simulink subsystem "VehicleElectroThermal"  (R2023a)
settings: Solver=VariableStepAuto  StartTime=0.0  StopTime=10.0  RelTol=1e-3
undefined symbols (not defined in the file): battery, cabin_T_init, coolant_pipe_D, coolant_valve_D_ratio_max, coolant_valve_D_ratio_min, coolant_valve_displacement, vehicleThermal
libraries: fl_lib x199, nesl_utility x54, SimscapeFluids_lib x15, ee_lib x9, sdl_lib x8, slpidlib x3, simulink x2, EmotorLib x2, BatteryCurrentManagement x1
(part 4 of 6)

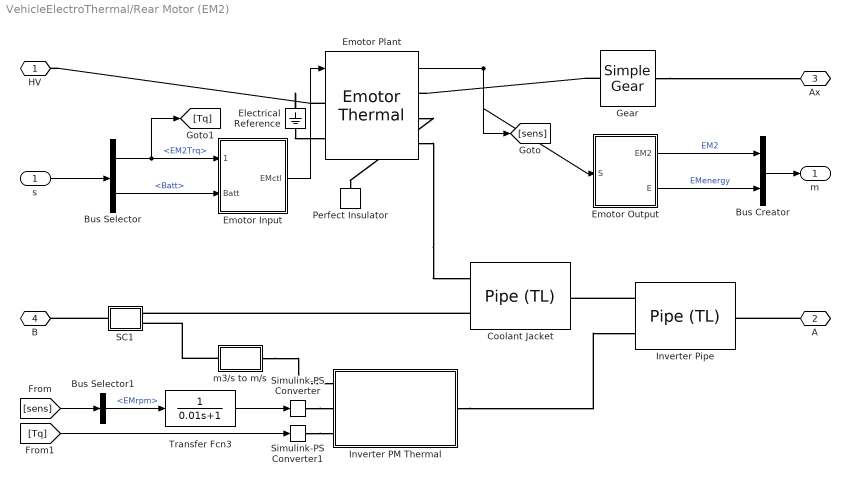
== system VehicleElectroThermal/Rear Motor (EM2) ==
  s : Inport
  Bus Creator : BusCreator  Inputs=2
  Bus Selector : BusSelector  OutputSignals=EM2Trq,Batt
  Bus Selector1 : BusSelector  OutputSignals=EMrpm
  Coolant Jacket : SimscapeFluids_lib/Thermal Liquid/Pipes & Fittings/Pipe (TL)  dynamic_compressibility=1  inertia=0  num_segments=1  pipe_length=0.4 m  cross_section_geometry=fluids.thermal_liquid.pipes_fittings.enum.CrossSectionGeometry.Custom  pipe_diameter=0.1 m  pipe_inner_diameter=0.05 m  pipe_outer_diameter=0.1 m  pipe_width=0.1 m  pipe_height=0.1 m  pipe_major_axis=0.1 m  pipe_minor_axis=0.05 m  pipe_side=0.1 m  pipe_angle=30 deg  area=4 * pi * vehicleThermal.coolant_channel_D^2 / 4 m^2  Dh=vehicleThermal.coolant_channel_D m  wall_spec=1  wall_compliance=1.2e-6 m/MPa  wall_time_constant=0.01 s  elevation_spec=foundation.enum.constant_variable.constant  elevation_gain=0 m  g=9.81 m/s^2  pressure_loss_spec=1  local_pressure_loss_spec=fluids.thermal_liquid.pipes_fittings.enum.LocalLossSpec.AggregateLength  length_add=20 * vehicleThermal.coolant_channel_D * 4 m  loss_coefficient=0.1  roughness_spec=fluids.thermal_liquid.pipes_fittings.enum.RoughnessSpec.Custom  roughness=1.5e-5 m  Re_friction_TLU=[ 400 1000 1.5e+3 3e+3 4e+3 6e+3 1e+4 2e+4 4e+4 6e+4 1e+5 1e+8 ]  friction_factor_TLU=[ 0.264 0.112 0.07099999999999999 0.0417 0.0387 0.0268 0.025 0.0232 0.0226 0.022 0.0214 0.0214 ]  shape_factor=64  Re_lam=100  Re_tur=500  mdot_nominal=[ 0.1 1 ] kg/s  p_diff_nominal=[ 0.001 0.01 ] MPa  mdot_threshold=1e-6 kg/s  heat_transfer_spec=4  mdot_nominal_heat=[ 0.1 1 ] kg/s  T_in_nominal=[ 293.15 293.15 ] K  T_out_nominal=[ 300 300 ] K  p_in_nominal_heat=[ 0.101325 0.101325 ] MPa  T_wall_nominal=[ 303.15 303.15 ] K  a_coeff=0.3  b_Re_power=0.8  c_Pr_power=0.33  Nu_lam=3.66  Re_Colburn_TLU=[ 100 150 1000 ]  Colburn_factor_TLU=[ 0.019 0.013 0.002 ]  Re_Nu_TLU=[ 100 150 1000 ]  Pr_Nu_TLU=[ 1 10 ]  Nu_TLU=[ 3.72 4.21; 3.75 4.44; 4.21 7.15 ]  p0_vec=vehicleThermal.coolant_p_init MPa  T0_vec=vehicleThermal.coolant_T_init K  mdot0=0.1 kg/s
  Electrical Reference : fl_lib/Electrical/Electrical Elements/Electrical Reference
  Emotor Input : Subsystem
  Emotor Output : Subsystem
  Emotor Plant : EmotorLib/Emotor Thermal  InitTemp=vehicleThermal.coolant_T_init  IronSpHeat=electricDrive.IronSpHeat  CopperSpHeat=electricDrive.CopperSpHeat  IronThConductivity=electricDrive.IronThConductivity  GrossToothMass=electricDrive.MotorThermal.GrossToothMass  WindingMass=electricDrive.MotorThermal.WindingMass  max_torque=electricDrive.max_torque  max_power=electricDrive.max_power  Tctc=electricDrive.Tctc  spMat=electricDrive.motor_loss_map.spMat  tqMat=electricDrive.motor_loss_map.tqMat  lossMat=electricDrive.motor_loss_map.lossMat  StatorBackIronMass=electricDrive.MotorThermal.StatorBackIronMass  StatorRootDia=electricDrive.MotorThermal.StatorRootDia  stator_od=electricDrive.MotorThermal.stator_od  StatorWindingOhArea=electricDrive.MotorThermal.StatorWindingOhArea  Bridgemass=electricDrive.MotorThermal.Bridgemass  rotor_od=electricDrive.MotorThermal.rotor_od  rotorStackLength=electricDrive.MotorThermal.rotorStackLength  RotorBackIronMass=electricDrive.MotorThermal.RotorBackIronMass  RotorAreaER=electricDrive.MotorThermal.RotorAreaER  RotorAreaCyl=electricDrive.MotorThermal.RotorAreaCyl
  Gear : sdl_lib/Gears/Simple Gear  ratio=10/3  rotation_direction=sdl.enum.shaftOutputDirection.same  friction_model=sdl.enum.gear_efficiencies_load.off  T_noload=0.1 N*m  T_nom=5 N*m  efficiency_nom=0.8  efficiency=0.8  temperature_TLU=[280, 300, 320] K  load_TLU=[1, 5, 10] N*m  efficiency_TLU=[.95, .9, .85]  efficiency_TLU2=[.85, .8, .75; .95, .9, .85; .85, .8, .7]  w_thr=0.01 rad/s  pwr_thr=0.001 W  enable_backlash=false  hardstop_model=simscape.enum.hardstop.smooth  backlash_distance=1e-3 mm  r_base=0.1 m  transition=1e-4 mm  backlash_stiffness=1e7 N/m  backlash_damping=1e6 N*s/m  coeff_rest=0  v_tol=0.001 m/s  f_tol=0 N  mu_visc=[0, 0] N*m*s/rad  enable_faults=simscape.enum.onoff.off  efficiency_fault=0.05  external_fault=simscape.enum.onoff.off  temporal_fault=simscape.enum.onoff.off  fault_time=5 s  fault_angles=pi / 12 rad  report_fault=simscape.enum.assert.action.none  thermal_mass=50 J/K  temperature_specify=off  temperature_priority=High  temperature=300 K  temperature_nominal_specify=off  temperature_nominal_unit=K  temperature_nominal_value=1  x_backlash_specify=off  x_backlash_priority=None  x_backlash=0 mm  x_backlash_nominal_specify=off  x_backlash_nominal_unit=mm  x_backlash_nominal_value=1  f_hardstop_specify=off  f_hardstop_priority=None  f_hardstop=0 N  f_hardstop_nominal_specify=off  f_hardstop_nominal_unit=N  f_hardstop_nominal_value=1  v_backlash_specify=off  v_backlash_priority=None  v_backlash=0 m/s  v_backlash_nominal_specify=off  v_backlash_nominal_unit=m/s  v_backlash_nominal_value=1
  Inverter PM Thermal : Subsystem
  Inverter Pipe : SimscapeFluids_lib/Thermal Liquid/Pipes & Fittings/Pipe (TL)  dynamic_compressibility=1  inertia=0  num_segments=1  pipe_length=0.4 m  cross_section_geometry=fluids.thermal_liquid.pipes_fittings.enum.CrossSectionGeometry.Custom  pipe_diameter=0.1 m  pipe_inner_diameter=0.05 m  pipe_outer_diameter=0.1 m  pipe_width=0.1 m  pipe_height=0.1 m  pipe_major_axis=0.1 m  pipe_minor_axis=0.05 m  pipe_side=0.1 m  pipe_angle=30 deg  area=4 * pi * vehicleThermal.coolant_channel_D^2 / 4 m^2  Dh=vehicleThermal.coolant_channel_D m  wall_spec=1  wall_compliance=1.2e-6 m/MPa  wall_time_constant=0.01 s  elevation_spec=foundation.enum.constant_variable.constant  elevation_gain=0 m  g=9.81 m/s^2  pressure_loss_spec=1  local_pressure_loss_spec=fluids.thermal_liquid.pipes_fittings.enum.LocalLossSpec.AggregateLength  length_add=20 * vehicleThermal.coolant_channel_D * 4 m  loss_coefficient=0.1  roughness_spec=fluids.thermal_liquid.pipes_fittings.enum.RoughnessSpec.Custom  roughness=1.5e-5 m  Re_friction_TLU=[ 400 1000 1.5e+3 3e+3 4e+3 6e+3 1e+4 2e+4 4e+4 6e+4 1e+5 1e+8 ]  friction_factor_TLU=[ 0.264 0.112 0.07099999999999999 0.0417 0.0387 0.0268 0.025 0.0232 0.0226 0.022 0.0214 0.0214 ]  shape_factor=64  Re_lam=100  Re_tur=500  mdot_nominal=[ 0.1 1 ] kg/s  p_diff_nominal=[ 0.001 0.01 ] MPa  mdot_threshold=1e-6 kg/s  heat_transfer_spec=4  mdot_nominal_heat=[ 0.1 1 ] kg/s  T_in_nominal=[ 293.15 293.15 ] K  T_out_nominal=[ 300 300 ] K  p_in_nominal_heat=[ 0.101325 0.101325 ] MPa  T_wall_nominal=[ 303.15 303.15 ] K  a_coeff=0.3  b_Re_power=0.8  c_Pr_power=0.33  Nu_lam=3.66  Re_Colburn_TLU=[ 100 150 1000 ]  Colburn_factor_TLU=[ 0.019 0.013 0.002 ]  Re_Nu_TLU=[ 100 150 1000 ]  Pr_Nu_TLU=[ 1 10 ]  Nu_TLU=[ 3.72 4.21; 3.75 4.44; 4.21 7.15 ]  p0_vec=vehicleThermal.coolant_p_init MPa  T0_vec=vehicleThermal.coolant_T_init K  mdot0=0.1 kg/s
  Perfect Insulator : fl_lib/Thermal/Thermal Elements/Perfect Insulator  T_specify=off  T_priority=None  T=293.15 K  T_nominal_specify=off  T_nominal_unit=K  T_nominal_value=1
  SC1 : Subsystem
      mask Display: disp(get_param(gcb, 'Name'))
  Simulink-PS Converter : nesl_utility/Simulink-PS Converter  PhysicalDomain=network_engine_domain  SubClassName=ps_input  LeftPortType=input  RightPortType=output  PseudoPeriodic=off  Frequencies=[]  NoiseDistribution=none  NoiseParameters=[]  Unit=rpm  AffineConversion=off  FilteringAndDerivatives=provide  SimscapeFilterOrder=1  InputFilterTimeConstant=0.001  UdotUserProvided=0
  Simulink-PS Converter1 : nesl_utility/Simulink-PS Converter  PhysicalDomain=network_engine_domain  SubClassName=ps_input  LeftPortType=input  RightPortType=output  PseudoPeriodic=off  Frequencies=[]  NoiseDistribution=none  NoiseParameters=[]  Unit=N*m  AffineConversion=off  FilteringAndDerivatives=provide  SimscapeFilterOrder=1  InputFilterTimeConstant=0.001  UdotUserProvided=0
  Transfer Fcn3 : TransferFcn  Denominator=[0.01 1]
  m3/s to m/s : Subsystem
  HV : PMIOPort  Side=Left
  A : PMIOPort  Port=2  Side=Left
  Ax : PMIOPort  Port=3  Side=Right
  B : PMIOPort  Port=4  Side=Right
  m : Outport
  wires:
  Transfer Fcn3/1 -> Simulink-PS Converter/1
  Bus Selector1/1 -> Transfer Fcn3/1  "<EMrpm>"
  [sens] -> Bus Selector1/1
  [Tq] -> Simulink-PS Converter1/1
  s/1 -> Bus Selector/1
  Emotor Output/2(E) -> Bus Creator/2  "EMenergy"
  Emotor Output/1(EM2) -> Bus Creator/1  "EM2"
  Bus Creator/1 -> m/1
  Emotor Input/1(EMctl) -> Emotor Plant/1
  Emotor Plant/1 -> [sens], Emotor Output/1(S)
  Bus Selector/2 -> Emotor Input/2(" Batt")  "<Batt>"
  Bus Selector/1 -> Emotor Input/1(TrqCmd), [Tq]  "<EM2Trq>"
  connections:
  Electrical Reference/LConn1 -- Emotor Plant/LConn2
  Gear/RConn1 -- Ax/RConn1
  Emotor Plant/RConn2 -- Perfect Insulator/LConn1
  Simulink-PS Converter/RConn1 -- Inverter PM Thermal/LConn2
  m3/s to m/s/LConn1 -- SC1/RConn2
  Emotor Plant/RConn3 -- Coolant Jacket/LConn2
  A/RConn1 -- Inverter Pipe/RConn1
  Coolant Jacket/LConn1 -- SC1/RConn1
  Inverter PM Thermal/RConn1 -- Inverter Pipe/LConn2
  SC1/LConn1 -- B/RConn1
  Simulink-PS Converter1/RConn1 -- Inverter PM Thermal/LConn3
  m3/s to m/s/RConn1 -- Inverter PM Thermal/LConn1
  Inverter Pipe/LConn1 -- Coolant Jacket/RConn1
  Emotor Plant/LConn1 -- HV/RConn1
  Gear/LConn1 -- Emotor Plant/RConn1

== system VehicleElectroThermal/Battery Pump/Pump Demand ==
  No current : fl_lib/Physical Signals/Sources/PS Constant  constant=0 A
  PS Abs : fl_lib/Physical Signals/Nonlinear Operators/PS Abs
      settings: InternalSimscapePortConfiguration="{\"Bottom\":[],\"Left\":[{\"id\":\"I\",\"label\":\"\",\"type\":\"input\"}],\"Right\":[{\"id\":\"O\",\"label\":\"\",\"type\":\"output\"}],\"Top\":[]}"
  PS Divide : fl_lib/Physical Signals/Functions/PS Divide
  PS Product : fl_lib/Physical Signals/Functions/PS Product
  PS Switch : fl_lib/Physical Signals/Nonlinear Operators/PS Switch  Threshold=0.5
      settings: InternalSimscapePortConfiguration="{\"Bottom\":[],\"Left\":[{\"id\":\"I1\",\"label\":\"\",\"type\":\"input\"},{\"id\":\"I2\",\"label\":\"\",\"type\":\"input\"},{\"id\":\"I3\",\"label\":\"\",\"type\":\"input\"}],\"Right\":[{\"id\":\"O\",\"label\":\"\",\"type\":\"output\"}],\"Top\":[]}"
  PS Switch1 : fl_lib/Physical Signals/Nonlinear Operators/PS Switch  Threshold=0.5
      settings: InternalSimscapePortConfiguration="{\"Bottom\":[],\"Left\":[{\"id\":\"I1\",\"label\":\"\",\"type\":\"input\"},{\"id\":\"I2\",\"label\":\"\",\"type\":\"input\"},{\"id\":\"I3\",\"label\":\"\",\"type\":\"input\"}],\"Right\":[{\"id\":\"O\",\"label\":\"\",\"type\":\"output\"}],\"Top\":[]}"
  Zero Divide Protection : fl_lib/Physical Signals/Sources/PS Constant  constant=1 V
  BatSt : PMIOPort  Side=Left
  Volt : PMIOPort  Port=2  Side=Left
  Q : PMIOPort  Port=3  Side=Left
  P : PMIOPort  Port=4  Side=Left
  I : PMIOPort  Port=5  Side=Right
  connections:
  PS Product/LConn2 -- PS Abs/RConn1
  Zero Divide Protection/RConn1 -- PS Switch1/LConn3
  PS Switch1/RConn1 -- PS Divide/LConn2
  PS Abs/LConn1 -- P/RConn1
  Q/RConn1 -- PS Product/LConn1
  PS Divide/LConn1 -- PS Product/RConn1
  PS Switch/RConn1 -- I/RConn1
  PS Switch1/LConn2 -- PS Switch/LConn2 -- BatSt/RConn1
  PS Switch/LConn1 -- PS Divide/RConn1
  PS Switch1/LConn1 -- Volt/RConn1
  No current/RConn1 -- PS Switch/LConn3

== system VehicleElectroThermal/Battery Pump/current sensing1 ==
  Current Sensor : fl_lib/Electrical/Electrical Sensors/Current Sensor
  PS-Simulink Converter : nesl_utility/PS-Simulink Converter  PhysicalDomain=network_engine_domain  SubClassName=ps_output  LeftPortType=input  RightPortType=output  PseudoPeriodic=off  Frequencies=[]  VectorFormat=inherit  Unit=inherit  AffineConversion=off
  "  " : PMIOPort  Side=Left
  " " : PMIOPort  Port=2  Side=Right
  "   " : Outport
  wires:
  PS-Simulink Converter/1 -> "   "/1
  connections:
  Current Sensor/RConn2 -- " "/RConn1
  Current Sensor/LConn1 -- "  "/RConn1
  PS-Simulink Converter/LConn1 -- Current Sensor/RConn1

== system VehicleElectroThermal/Chiller/Chiller Subsystem ==
  BattSt : Inport
  ThCtrl : Inport  Port=2
  Chiller Demand : Subsystem
  Compare To Constant : simulink/Logic and Bit Operations/Compare To Constant  relop=>  const=0  OutDataTypeStr=boolean
  Constant1 : Constant  Value=0
  Constant2 : Constant
  Max Power [W] : Gain  Gain=-vehicleThermal.chillerMaxPower
  Product : Product
  Simulink-PS Converter : nesl_utility/Simulink-PS Converter  PhysicalDomain=network_engine_domain  SubClassName=ps_input  LeftPortType=input  RightPortType=output  PseudoPeriodic=off  Frequencies=[]  NoiseDistribution=none  NoiseParameters=[]  Unit=W  AffineConversion=off  FilteringAndDerivatives=provide  SimscapeFilterOrder=1  InputFilterTimeConstant=0.001  UdotUserProvided=0
  Simulink-PS Converter2 : nesl_utility/Simulink-PS Converter  PhysicalDomain=network_engine_domain  SubClassName=ps_input  LeftPortType=input  RightPortType=output  PseudoPeriodic=off  Frequencies=[]  NoiseDistribution=none  NoiseParameters=[]  Unit=1  AffineConversion=off  FilteringAndDerivatives=provide  SimscapeFilterOrder=1  InputFilterTimeConstant=0.001  UdotUserProvided=0
  Switch : Switch  Criteria=u2 > Threshold  SaturateOnIntegerOverflow=off  InputSameDT=off
  Transfer Fcn : TransferFcn  Denominator=[1 1]
  V : PMIOPort  Side=Left
  I : PMIOPort  Port=2  Side=Right
  output : PMIOPort  Port=3  Side=Right
  wires:
  Constant1/1 -> Switch/1
  Constant2/1 -> Switch/3
  Compare To Constant/1 -> Product/1
  Product/1 -> Simulink-PS Converter/1
  BattSt/1 -> Simulink-PS Converter2/1, Compare To Constant/1
  Transfer Fcn/1 -> Max Power [W]/1
  ThCtrl/1 -> Switch/2
  Switch/1 -> Transfer Fcn/1
  Max Power [W]/1 -> Product/2
  connections:
  Chiller Demand/RConn1 -- I/RConn1
  Chiller Demand/LConn2 -- Simulink-PS Converter2/RConn1
  Chiller Demand/LConn1 -- V/RConn1
  Chiller Demand/LConn3 -- output/RConn1 -- Simulink-PS Converter/RConn1

== system VehicleElectroThermal/Chiller/current sensing1 ==
  Current Sensor : fl_lib/Electrical/Electrical Sensors/Current Sensor
  PS-Simulink Converter : nesl_utility/PS-Simulink Converter  PhysicalDomain=network_engine_domain  SubClassName=ps_output  LeftPortType=input  RightPortType=output  PseudoPeriodic=off  Frequencies=[]  VectorFormat=inherit  Unit=inherit  AffineConversion=off
  "  " : PMIOPort  Side=Left
  " " : PMIOPort  Port=2  Side=Right
  "   " : Outport
  wires:
  PS-Simulink Converter/1 -> "   "/1
  connections:
  Current Sensor/RConn2 -- " "/RConn1
  Current Sensor/LConn1 -- "  "/RConn1
  PS-Simulink Converter/LConn1 -- Current Sensor/RConn1

== system VehicleElectroThermal/Chiller Bypass Valve/Valve Control ==
  ThCtrl : Inport
  Bias : Bias  Bias=-1  SaturateOnIntegerOverflow=off
  Gain : Gain  Gain=2
  Max Valve Displacement [m] : Gain  Gain=vehicleThermal.coolant_valve_displacement
  Simulink-PS Converter : nesl_utility/Simulink-PS Converter  PhysicalDomain=network_engine_domain  SubClassName=ps_input  LeftPortType=input  RightPortType=output  PseudoPeriodic=off  Frequencies=[]  NoiseDistribution=none  NoiseParameters=[]  Unit=m  AffineConversion=off  FilteringAndDerivatives=provide  SimscapeFilterOrder=1  InputFilterTimeConstant=0.001  UdotUserProvided=0
  Transfer Fcn : TransferFcn  Denominator=[1 1]
  Disp : PMIOPort  Side=Right
  wires:
  Transfer Fcn/1 -> Gain/1
  ThCtrl/1 -> Transfer Fcn/1
  Max Valve Displacement [m]/1 -> Simulink-PS Converter/1
  Bias/1 -> Max Valve Displacement [m]/1
  Gain/1 -> Bias/1
  connections:
  Simulink-PS Converter/RConn1 -- Disp/RConn1

== system VehicleElectroThermal/Front Motor (EM1)/Emotor Input ==
  "Tq  " : Inport
  "Batt " : Inport  Port=2
  Bus Creator : BusCreator  Inputs=3
  Bus Selector3 : BusSelector  OutputSignals=Relay.RelayDchg,BattSensor.BatVolt
  Constant : Constant
  Constant1 : Constant  Value=0
  Gain : Gain
  Switch : Switch  Criteria=u2 > Threshold  SaturateOnIntegerOverflow=off  InputSameDT=off
  EMctl : Outport
  wires:
  Gain/1 -> Bus Creator/3  "BatVolt"
  Bus Selector3/2 -> Gain/1  "<BatVolt>"
  Bus Creator/1 -> EMctl/1
  "Batt "/1 -> Bus Selector3/1
  Bus Selector3/1 -> Switch/2  "<RelayDchg>"
  Constant/1 -> Switch/3
  Constant1/1 -> Switch/1
  Switch/1 -> Bus Creator/2  "fault"
  "Tq  "/1 -> Bus Creator/1  "EMtrq"

== system VehicleElectroThermal/Front Motor (EM1)/Emotor Output ==
  S : Inport
  Bus Selector1 : BusSelector  OutputSignals=Current,Volt
  Constant : Constant  Value=3600
  Divide : Product  Inputs=*/
  Integrator : Integrator
  Product : Product
  EM : Outport
  E : Outport  Port=2
  wires:
  Bus Selector1/1 -> Product/1  "<Current>"
  Bus Selector1/2 -> Product/2  "<Volt>"
  S/1 -> Bus Selector1/1, EM/1  "EMsensor"
  Product/1 -> Integrator/1
  Integrator/1 -> Divide/1
  Constant/1 -> Divide/2
  Divide/1 -> E/1  "EMenergy"

== system VehicleElectroThermal/Front Motor (EM1)/Inverter PM Thermal ==
  IGBTlossTable : fl_lib/Physical Signals/Lookup Tables/PS Lookup Table (3D)  x1=electricDrive.motor_loss_map.spMat rpm  x2=electricDrive.motor_loss_map.tqMat N*m  x3=[25,125, 175]+273.15 K  f=electricDrive.inverter_loss_map.lossMatIgbt  interp_method=simscape.enum.interpolation.linear  extrap_method=simscape.enum.extrapolation.linear
      settings: InternalSimscapePortConfiguration="{\"Bottom\":[],\"Left\":[{\"id\":\"I1\",\"label\":\"x1\",\"type\":\"input\"},{\"id\":\"I2\",\"label\":\"x2\",\"type\":\"input\"},{\"id\":\"I3\",\"label\":\"x3\",\"type\":\"input\"}],\"Right\":[{\"id\":\"O\",\"label\":\"f\",\"type\":\"output\"}],\"Top\":[]}"
  PM Cauer thermall : Subsystem
      settings: PortSchema="{\"entries\":[{\"content\":{\"sides\":[{\"content\":{\"connectorIds\":[\"LConn1\"]},\"type\":\"ConnectorPlacement.EquallySpacedRectSide\",\"uuid\":\"c466717f-a559-4c42-b6dd-2de508982627\"},{\"content\":{\"connectorIds\":[\"RConn1\",\"RConn2\",\"RConn3\"],\"side\":\"RIGHT\"},\"type\":\"ConnectorPlacement.EquallySpacedRectSide\",\"uuid\":\"5a44429a-0c01-47a4-96c4-89a03d92af2a\"},{\"content\":{\"connectorIds\":[],\"side\":\"TOP\"},\"type\":\"ConnectorPlacement.EquallySpacedRectSide\",\"uuid\":\"592797f6-2176-45a1-8a5a-ffba72eaaa30\"},{\"content\":{\"connectorIds\":[\"RConn4\",\"RConn5\"],\"side\":\"BOTTOM\"},\"type\":\"ConnectorPlacement.EquallySpacedRectSide\",\"uuid\":\"45f39216-5c54-48d4-857b-159bfbffda40\"}]},\"type\":\"ConnectorPlacement.EquallySpacedConnector\",\"uuid\":\"8211d252-7bec-4c59-be39-60a0fcf206ce\"}],\"packageUris\":[\"http://schema.mathworks.com/mf0/Connector/R2020b\"],\"version\":\"1.0\"}"
  PS Gain : fl_lib/Physical Signals/Functions/PS Gain  gain=6 J/s
  PS Gain1 : fl_lib/Physical Signals/Functions/PS Gain  gain=6 J/s
  diodeLossTable : fl_lib/Physical Signals/Lookup Tables/PS Lookup Table (3D)  x1=electricDrive.motor_loss_map.spMat rpm  x2=electricDrive.motor_loss_map.tqMat N*m  x3=[25,125, 175]+273.15 K  f=electricDrive.inverter_loss_map.lossMatDiode  interp_method=simscape.enum.interpolation.linear  extrap_method=simscape.enum.extrapolation.linear
      settings: InternalSimscapePortConfiguration="{\"Bottom\":[],\"Left\":[{\"id\":\"I1\",\"label\":\"x1\",\"type\":\"input\"},{\"id\":\"I2\",\"label\":\"x2\",\"type\":\"input\"},{\"id\":\"I3\",\"label\":\"x3\",\"type\":\"input\"}],\"Right\":[{\"id\":\"O\",\"label\":\"f\",\"type\":\"output\"}],\"Top\":[]}"
  Vliq : PMIOPort  Side=Left
  Motor RPM : PMIOPort  Port=2  Side=Left
  Motor Torque : PMIOPort  Port=3  Side=Left
  H : PMIOPort  Port=4  Side=Right
  connections:
  PS Gain1/RConn1 -- PM Cauer thermall/RConn3
  PS Gain/RConn1 -- PM Cauer thermall/RConn1
  PM Cauer thermall/RConn5 -- IGBTlossTable/LConn3
  PM Cauer thermall/RConn2 -- diodeLossTable/LConn3
  diodeLossTable/LConn2 -- IGBTlossTable/LConn2 -- Motor Torque/RConn1
  diodeLossTable/LConn1 -- Motor RPM/RConn1 -- IGBTlossTable/LConn1
  Vliq/RConn1 -- PM Cauer thermall/RConn4
  diodeLossTable/RConn1 -- PS Gain/LConn1
  IGBTlossTable/RConn1 -- PS Gain1/LConn1
  H/RConn1 -- PM Cauer thermall/LConn1

== system VehicleElectroThermal/Front Motor (EM1)/SC1 ==
  Absolute Reference (TL) : fl_lib/Thermal Liquid/Elements/Absolute Reference (TL)
  Pressure & Temperature Sensor (TL) : fl_lib/Thermal Liquid/Sensors/Pressure & Temperature Sensor (TL)  reference=foundation.enum.MeasurementReference.difference  pressure=true  pressure_spec=foundation.enum.PressureMeasementSpec.Absolute  temperature=true
      settings: InternalSimscapePortConfiguration="{\"Bottom\":[{\"id\":\"T\",\"label\":\"T\",\"type\":\"output\"}],\"Left\":[{\"id\":\"A\",\"label\":\"A\",\"type\":\"foundation.thermal_liquid.thermal_liquid\"}],\"Right\":[{\"id\":\"B\",\"label\":\"B\",\"type\":\"foundation.thermal_liquid.thermal_liquid\"},{\"id\":\"P\",\"label\":\"P\",\"type\":\"output\"}],\"Top\":[]}"
  Volumetric Flow Rate Sensor (TL) : fl_lib/Thermal Liquid/Sensors/Flow Rate Sensor (TL)  mass_flow_measure=false  volumetric_flow_measure=true  energy_flow_measure=false
      settings: InternalSimscapePortConfiguration="{\"Bottom\":[],\"Left\":[{\"id\":\"A\",\"label\":\"A\",\"type\":\"foundation.thermal_liquid.thermal_liquid\"}],\"Right\":[{\"id\":\"B\",\"label\":\"B\",\"type\":\"foundation.thermal_liquid.thermal_liquid\"},{\"id\":\"V\",\"label\":\"V\",\"type\":\"output\"}],\"Top\":[]}"
  B : PMIOPort  Side=Left
  A : PMIOPort  Port=2  Side=Right
  m3/s : PMIOPort  Port=3  Side=Right
  connections:
  Volumetric Flow Rate Sensor (TL)/RConn2 -- m3/s/RConn1
  Absolute Reference (TL)/LConn1 -- Pressure & Temperature Sensor (TL)/RConn1
  Volumetric Flow Rate Sensor (TL)/LConn1 -- B/RConn1
  A/RConn1 -- Volumetric Flow Rate Sensor (TL)/RConn1 -- Pressure & Temperature Sensor (TL)/LConn1

== system VehicleElectroThermal/Front Motor (EM1)/TempSens ==
  Absolute Reference (TL) : fl_lib/Thermal Liquid/Elements/Absolute Reference (TL)
  PS-Simulink Converter7 : nesl_utility/PS-Simulink Converter  PhysicalDomain=network_engine_domain  SubClassName=ps_output  LeftPortType=input  RightPortType=output  PseudoPeriodic=off  Frequencies=[]  VectorFormat=inherit  Unit=inherit  AffineConversion=off
  Pressure & Temperature Sensor (TL) : fl_lib/Thermal Liquid/Sensors/Pressure & Temperature Sensor (TL)  reference=foundation.enum.MeasurementReference.difference  pressure=true  pressure_spec=foundation.enum.PressureMeasementSpec.Absolute  temperature=true
      settings: InternalSimscapePortConfiguration="{\"Bottom\":[{\"id\":\"T\",\"label\":\"T\",\"type\":\"output\"}],\"Left\":[{\"id\":\"A\",\"label\":\"A\",\"type\":\"foundation.thermal_liquid.thermal_liquid\"}],\"Right\":[{\"id\":\"B\",\"label\":\"B\",\"type\":\"foundation.thermal_liquid.thermal_liquid\"},{\"id\":\"P\",\"label\":\"P\",\"type\":\"output\"}],\"Top\":[]}"
  " " : PMIOPort  Side=Left
  "  " : Outport
  wires:
  PS-Simulink Converter7/1 -> "  "/1
  connections:
  Pressure & Temperature Sensor (TL)/LConn1 -- " "/RConn1
  Absolute Reference (TL)/LConn1 -- Pressure & Temperature Sensor (TL)/RConn1
  Pressure & Temperature Sensor (TL)/RConn3 -- PS-Simulink Converter7/LConn1

== system VehicleElectroThermal/Front Motor (EM1)/m3//s to m//s ==
  note: Q=Av
  Coolant Area : fl_lib/Physical Signals/Sources/PS Constant  constant=4 * pi * vehicleThermal.coolant_channel_D^2 / 4 m^2
  PS Divide : fl_lib/Physical Signals/Functions/PS Divide
  PS Saturation : fl_lib/Physical Signals/Nonlinear Operators/PS Saturation  upper_limit=10 m/s  lower_limit=1e-6 m/s
  "  " : PMIOPort  Side=Left
  Vliq : PMIOPort  Port=2  Side=Right
  connections:
  PS Saturation/RConn1 -- Vliq/RConn1
  PS Divide/RConn1 -- PS Saturation/LConn1
  "  "/RConn1 -- PS Divide/LConn1
  PS Divide/LConn2 -- Coolant Area/RConn1

== system VehicleElectroThermal/HVAC/Cabin ==
  Tenv : Inport
  Tsetpoint : Inport  Port=2
  acOnOff : Inport  Port=3
  Cabin Control : Subsystem
  Cabin Plant : Subsystem
  Cool : Outport
  PTC : Outport  Port=2
  wires:
  acOnOff/1 -> Cabin Control/6(acOnOff)
  Tenv/1 -> Cabin Plant/1(EnvTp), Cabin Control/1(Tenv)
  Tsetpoint/1 -> Cabin Control/5(Tsetpoint)
  [Tcabin] -> Cabin Control/3(Tcabin)
  [TacVent] -> Cabin Control/4(TacVent)
  Cabin Control/3(cmdCool) -> Cool/1, Cabin Plant/4(cmdCool)
  [Tptc] -> Cabin Control/2(Tptc)
  Cabin Plant/3(cabinTp) -> [Tcabin]
  Cabin Plant/2(CoolerTp) -> [TacVent]
  Cabin Control/1(cmdBlower) -> Cabin Plant/2(cmdBlower)
  Cabin Control/2(PTC) -> Cabin Plant/3(cmdPTC), PTC/1
  Cabin Plant/1(ptcTp) -> [Tptc]

== system VehicleElectroThermal/HVAC/HVAC Demand ==
  Display : Display
  Display1 : Display
  Display2 : Display
  No current : fl_lib/Physical Signals/Sources/PS Constant  constant=0 A
  PS Abs : fl_lib/Physical Signals/Nonlinear Operators/PS Abs
      settings: InternalSimscapePortConfiguration="{\"Bottom\":[],\"Left\":[{\"id\":\"I\",\"label\":\"\",\"type\":\"input\"}],\"Right\":[{\"id\":\"O\",\"label\":\"\",\"type\":\"output\"}],\"Top\":[]}"
  PS Add : fl_lib/Physical Signals/Functions/PS Add
  PS Add1 : fl_lib/Physical Signals/Functions/PS Add
  PS Divide : fl_lib/Physical Signals/Functions/PS Divide
  PS Switch : fl_lib/Physical Signals/Nonlinear Operators/PS Switch  Threshold=0.5
      settings: InternalSimscapePortConfiguration="{\"Bottom\":[],\"Left\":[{\"id\":\"I1\",\"label\":\"\",\"type\":\"input\"},{\"id\":\"I2\",\"label\":\"\",\"type\":\"input\"},{\"id\":\"I3\",\"label\":\"\",\"type\":\"input\"}],\"Right\":[{\"id\":\"O\",\"label\":\"\",\"type\":\"output\"}],\"Top\":[]}"
  PS-Simulink Converter : nesl_utility/PS-Simulink Converter  PhysicalDomain=network_engine_domain  SubClassName=ps_output  LeftPortType=input  RightPortType=output  PseudoPeriodic=off  Frequencies=[]  VectorFormat=inherit  Unit=inherit  AffineConversion=off
  PS-Simulink Converter1 : nesl_utility/PS-Simulink Converter  PhysicalDomain=network_engine_domain  SubClassName=ps_output  LeftPortType=input  RightPortType=output  PseudoPeriodic=off  Frequencies=[]  VectorFormat=inherit  Unit=inherit  AffineConversion=off
  PS-Simulink Converter2 : nesl_utility/PS-Simulink Converter  PhysicalDomain=network_engine_domain  SubClassName=ps_output  LeftPortType=input  RightPortType=output  PseudoPeriodic=off  Frequencies=[]  VectorFormat=inherit  Unit=inherit  AffineConversion=off
  Zero Divide Protection : fl_lib/Physical Signals/Sources/PS Constant  constant=10 V
  Volt : PMIOPort  Side=Left
  BatSt : PMIOPort  Port=2  Side=Left
  Cool : PMIOPort  Port=3  Side=Left
  I : PMIOPort  Port=4  Side=Right
  PTC : PMIOPort  Port=5  Side=Left
  wires:
  PS-Simulink Converter/1 -> Display2/1
  PS-Simulink Converter2/1 -> Display1/1
  PS-Simulink Converter1/1 -> Display/1
  connections:
  Volt/RConn1 -- PS Add1/LConn1
  PS-Simulink Converter1/LConn1 -- PS Divide/LConn1 -- PS Add/RConn1
  PTC/RConn1 -- PS Add/LConn2
  Cool/RConn1 -- PS Abs/LConn1
  PS Abs/RConn1 -- PS Add/LConn1
  PS Add1/LConn2 -- Zero Divide Protection/RConn1
  PS-Simulink Converter/LConn1 -- PS Add1/RConn1 -- PS Divide/LConn2
  PS Switch/RConn1 -- I/RConn1
  BatSt/RConn1 -- PS Switch/LConn2
  PS Divide/RConn1 -- PS Switch/LConn1 -- PS-Simulink Converter2/LConn1
  No current/RConn1 -- PS Switch/LConn3

== system VehicleElectroThermal/HVAC/HVAC Energy ==
  I : Inport
  Batt : Inport  Port=2
  Bus Selector : BusSelector  OutputSignals=BattSensor.BatVolt
  Constant : Constant  Value=3600
  Divide : Product  Inputs=*/
  Integrator : Integrator
  Product : Product
  E : Outport
  wires:
  Bus Selector/1 -> Product/2  "<BatVolt>"
  Product/1 -> Integrator/1
  Integrator/1 -> Divide/1
  Constant/1 -> Divide/2
  Batt/1 -> Bus Selector/1
  Divide/1 -> E/1
  I/1 -> Product/1

== system VehicleElectroThermal/Heater/Heater Subsystem ==
  Batt : Inport
  ThCtrl : Inport  Port=2
  Compare To Constant : simulink/Logic and Bit Operations/Compare To Constant  relop=>  const=0  OutDataTypeStr=boolean
  Heater Demand : Subsystem
  Max Power [W] : Gain  Gain=vehicleThermal.heaterMaxPower
  Product : Product
  Simulink-PS Converter : nesl_utility/Simulink-PS Converter  PhysicalDomain=network_engine_domain  SubClassName=ps_input  LeftPortType=input  RightPortType=output  PseudoPeriodic=off  Frequencies=[]  NoiseDistribution=none  NoiseParameters=[]  Unit=W  AffineConversion=off  FilteringAndDerivatives=provide  SimscapeFilterOrder=1  InputFilterTimeConstant=0.001  UdotUserProvided=0
  Simulink-PS Converter2 : nesl_utility/Simulink-PS Converter  PhysicalDomain=network_engine_domain  SubClassName=ps_input  LeftPortType=input  RightPortType=output  PseudoPeriodic=off  Frequencies=[]  NoiseDistribution=none  NoiseParameters=[]  Unit=1  AffineConversion=off  FilteringAndDerivatives=provide  SimscapeFilterOrder=1  InputFilterTimeConstant=0.001  UdotUserProvided=0
  Transfer Fcn : TransferFcn  Denominator=[1 1]
  V : PMIOPort  Side=Left
  I : PMIOPort  Port=2  Side=Right
  output : PMIOPort  Port=3  Side=Right
  wires:
  Batt/1 -> Simulink-PS Converter2/1, Compare To Constant/1
  ThCtrl/1 -> Transfer Fcn/1
  Compare To Constant/1 -> Product/1
  Max Power [W]/1 -> Product/2
  Transfer Fcn/1 -> Max Power [W]/1
  Product/1 -> Simulink-PS Converter/1
  connections:
  Heater Demand/RConn1 -- I/RConn1
  Heater Demand/LConn2 -- Simulink-PS Converter2/RConn1
  Heater Demand/LConn1 -- V/RConn1
  output/RConn1 -- Heater Demand/LConn3 -- Simulink-PS Converter/RConn1

== system VehicleElectroThermal/Heater/current sensing1 ==
  Current Sensor : fl_lib/Electrical/Electrical Sensors/Current Sensor
  PS-Simulink Converter : nesl_utility/PS-Simulink Converter  PhysicalDomain=network_engine_domain  SubClassName=ps_output  LeftPortType=input  RightPortType=output  PseudoPeriodic=off  Frequencies=[]  VectorFormat=inherit  Unit=inherit  AffineConversion=off
  "  " : PMIOPort  Side=Left
  " " : PMIOPort  Port=2  Side=Right
  "   " : Outport
  wires:
  PS-Simulink Converter/1 -> "   "/1
  connections:
  Current Sensor/RConn2 -- " "/RConn1
  Current Sensor/LConn1 -- "  "/RConn1
  PS-Simulink Converter/LConn1 -- Current Sensor/RConn1

== system VehicleElectroThermal/Motor Pump/Pump Demand ==
  No current : fl_lib/Physical Signals/Sources/PS Constant  constant=0 A
  PS Abs : fl_lib/Physical Signals/Nonlinear Operators/PS Abs
      settings: InternalSimscapePortConfiguration="{\"Bottom\":[],\"Left\":[{\"id\":\"I\",\"label\":\"\",\"type\":\"input\"}],\"Right\":[{\"id\":\"O\",\"label\":\"\",\"type\":\"output\"}],\"Top\":[]}"
  PS Divide : fl_lib/Physical Signals/Functions/PS Divide
  PS Product : fl_lib/Physical Signals/Functions/PS Product
  PS Switch : fl_lib/Physical Signals/Nonlinear Operators/PS Switch  Threshold=0.5
      settings: InternalSimscapePortConfiguration="{\"Bottom\":[],\"Left\":[{\"id\":\"I1\",\"label\":\"\",\"type\":\"input\"},{\"id\":\"I2\",\"label\":\"\",\"type\":\"input\"},{\"id\":\"I3\",\"label\":\"\",\"type\":\"input\"}],\"Right\":[{\"id\":\"O\",\"label\":\"\",\"type\":\"output\"}],\"Top\":[]}"
  PS Switch1 : fl_lib/Physical Signals/Nonlinear Operators/PS Switch  Threshold=0.5
      settings: InternalSimscapePortConfiguration="{\"Bottom\":[],\"Left\":[{\"id\":\"I1\",\"label\":\"\",\"type\":\"input\"},{\"id\":\"I2\",\"label\":\"\",\"type\":\"input\"},{\"id\":\"I3\",\"label\":\"\",\"type\":\"input\"}],\"Right\":[{\"id\":\"O\",\"label\":\"\",\"type\":\"output\"}],\"Top\":[]}"
  Zero Divide Protection : fl_lib/Physical Signals/Sources/PS Constant  constant=1 V
  BatSt : PMIOPort  Side=Left
  Volt : PMIOPort  Port=2  Side=Left
  Q : PMIOPort  Port=3  Side=Left
  P : PMIOPort  Port=4  Side=Left
  I : PMIOPort  Port=5  Side=Right
  connections:
  PS Abs/RConn1 -- PS Product/LConn2
  Zero Divide Protection/RConn1 -- PS Switch1/LConn3
  PS Switch1/RConn1 -- PS Divide/LConn2
  Q/RConn1 -- PS Product/LConn1
  P/RConn1 -- PS Abs/LConn1
  PS Divide/LConn1 -- PS Product/RConn1
  PS Switch/RConn1 -- I/RConn1
  PS Switch/LConn2 -- PS Switch1/LConn2 -- BatSt/RConn1
  PS Switch/LConn1 -- PS Divide/RConn1
  PS Switch1/LConn1 -- Volt/RConn1
  No current/RConn1 -- PS Switch/LConn3

== system VehicleElectroThermal/Motor Pump/current sensing1 ==
  Current Sensor : fl_lib/Electrical/Electrical Sensors/Current Sensor
  PS-Simulink Converter : nesl_utility/PS-Simulink Converter  PhysicalDomain=network_engine_domain  SubClassName=ps_output  LeftPortType=input  RightPortType=output  PseudoPeriodic=off  Frequencies=[]  VectorFormat=inherit  Unit=inherit  AffineConversion=off
  "  " : PMIOPort  Side=Left
  " " : PMIOPort  Port=2  Side=Right
  "   " : Outport
  wires:
  PS-Simulink Converter/1 -> "   "/1
  connections:
  Current Sensor/RConn2 -- " "/RConn1
  Current Sensor/LConn1 -- "  "/RConn1
  PS-Simulink Converter/LConn1 -- Current Sensor/RConn1

== system VehicleElectroThermal/Parallel-Serial Mode Valve/Battery Coolant Tank Heat Transfer ==
  Tenv : Inport
  Convective Heat Transfer : fl_lib/Thermal/Thermal Elements/Convective Heat Transfer  thermal_type=foundation.enum.constant_variable.constant  area=3 * vehicleThermal.coolant_tank_area m^2  heat_tr_coeff=20 W/(m^2 * K)  min_heat_tr_coeff=1e-3 W/(K*m^2)  T_specify=off  T_priority=None  T=0 K  T_nominal_specify=off  T_nominal_unit=K  T_nominal_value=1  Q_specify=off  Q_priority=None  Q=0 W  Q_nominal_specify=off  Q_nominal_unit=W  Q_nominal_value=1
  Convective Heat Transfer1 : fl_lib/Thermal/Thermal Elements/Convective Heat Transfer  thermal_type=foundation.enum.constant_variable.constant  area=3 * vehicleThermal.coolant_tank_area m^2  heat_tr_coeff=20 W/(m^2 * K)  min_heat_tr_coeff=1e-3 W/(K*m^2)  T_specify=off  T_priority=None  T=0 K  T_nominal_specify=off  T_nominal_unit=K  T_nominal_value=1  Q_specify=off  Q_priority=None  Q=0 W  Q_nominal_specify=off  Q_nominal_unit=W  Q_nominal_value=1
  Environment Temperature : fl_lib/Thermal/Thermal Sources/Controlled Temperature Source
  Simulink-PS Converter : nesl_utility/Simulink-PS Converter  PhysicalDomain=network_engine_domain  SubClassName=ps_input  LeftPortType=input  RightPortType=output  PseudoPeriodic=off  Frequencies=[]  NoiseDistribution=none  NoiseParameters=[]  Unit=K  AffineConversion=on  FilteringAndDerivatives=provide  SimscapeFilterOrder=1  InputFilterTimeConstant=0.001  UdotUserProvided=0
  Thermal Reference : fl_lib/Thermal/Thermal Elements/Thermal Reference
  A : PMIOPort  Side=Left
  B : PMIOPort  Port=2  Side=Left
  wires:
  Tenv/1 -> Simulink-PS Converter/1
  connections:
  Convective Heat Transfer/LConn1 -- A/RConn1
  B/RConn1 -- Convective Heat Transfer1/LConn1
  Simulink-PS Converter/RConn1 -- Environment Temperature/RConn1
  Thermal Reference/LConn1 -- Environment Temperature/RConn2
  Environment Temperature/LConn1 -- Convective Heat Transfer1/RConn1 -- Convective Heat Transfer/RConn1

== system VehicleElectroThermal/Parallel-Serial Mode Valve/Motor Coolant Tank Heat Transfer ==
  Tenv : Inport
  Convective Heat Transfer : fl_lib/Thermal/Thermal Elements/Convective Heat Transfer  thermal_type=foundation.enum.constant_variable.constant  area=3 * vehicleThermal.coolant_tank_area m^2  heat_tr_coeff=20 W/(m^2 * K)  min_heat_tr_coeff=1e-3 W/(K*m^2)  T_specify=off  T_priority=None  T=0 K  T_nominal_specify=off  T_nominal_unit=K  T_nominal_value=1  Q_specify=off  Q_priority=None  Q=0 W  Q_nominal_specify=off  Q_nominal_unit=W  Q_nominal_value=1
  Convective Heat Transfer1 : fl_lib/Thermal/Thermal Elements/Convective Heat Transfer  thermal_type=foundation.enum.constant_variable.constant  area=3 * vehicleThermal.coolant_tank_area m^2  heat_tr_coeff=20 W/(m^2 * K)  min_heat_tr_coeff=1e-3 W/(K*m^2)  T_specify=off  T_priority=None  T=0 K  T_nominal_specify=off  T_nominal_unit=K  T_nominal_value=1  Q_specify=off  Q_priority=None  Q=0 W  Q_nominal_specify=off  Q_nominal_unit=W  Q_nominal_value=1
  Environment Temperature : fl_lib/Thermal/Thermal Sources/Controlled Temperature Source
  Simulink-PS Converter : nesl_utility/Simulink-PS Converter  PhysicalDomain=network_engine_domain  SubClassName=ps_input  LeftPortType=input  RightPortType=output  PseudoPeriodic=off  Frequencies=[]  NoiseDistribution=none  NoiseParameters=[]  Unit=K  AffineConversion=on  FilteringAndDerivatives=provide  SimscapeFilterOrder=1  InputFilterTimeConstant=0.001  UdotUserProvided=0
  Thermal Reference : fl_lib/Thermal/Thermal Elements/Thermal Reference
  A : PMIOPort  Side=Right
  B : PMIOPort  Port=2  Side=Right
  wires:
  Tenv/1 -> Simulink-PS Converter/1
  connections:
  A/RConn1 -- Convective Heat Transfer/LConn1
  B/RConn1 -- Convective Heat Transfer1/LConn1
  Convective Heat Transfer1/RConn1 -- Environment Temperature/LConn1 -- Convective Heat Transfer/RConn1
  Thermal Reference/LConn1 -- Environment Temperature/RConn2
  Simulink-PS Converter/RConn1 -- Environment Temperature/RConn1

== system VehicleElectroThermal/Parallel-Serial Mode Valve/Valve Control ==
  Ctrl : Inport
  Bias : Bias  Bias=-1  SaturateOnIntegerOverflow=off
  Gain : Gain  Gain=2
  Max Valve Displacement [m] : Gain  Gain=vehicleThermal.coolant_valve_displacement
  Simulink-PS Converter : nesl_utility/Simulink-PS Converter  PhysicalDomain=network_engine_domain  SubClassName=ps_input  LeftPortType=input  RightPortType=output  PseudoPeriodic=off  Frequencies=[]  NoiseDistribution=none  NoiseParameters=[]  Unit=m  AffineConversion=off  FilteringAndDerivatives=provide  SimscapeFilterOrder=1  InputFilterTimeConstant=0.001  UdotUserProvided=0
  Transfer Fcn : TransferFcn  Denominator=[1 1]
  disp : PMIOPort  Side=Right
  wires:
  Ctrl/1 -> Transfer Fcn/1
  Max Valve Displacement [m]/1 -> Simulink-PS Converter/1
  Transfer Fcn/1 -> Gain/1
  Gain/1 -> Bias/1
  Bias/1 -> Max Valve Displacement [m]/1
  connections:
  Simulink-PS Converter/RConn1 -- disp/RConn1

== system VehicleElectroThermal/Radiator/Fan_Control ==
  VehSpd : Inport
  FanCtrl : Inport  Port=2
  Air Speed Table [m/s] : Lookup_n-D  BreakpointsForDimension1=[0 40 90 110 150 180 198]  BreakpointsForDimension2=[0 14.4]  IndexSearchMethod=Linear search  BeginIndexSearchUsingPreviousIndexResult=on  Table=[0 0.8 2.2 2.7 3.6 4.1 4.6; 1.5 2.3 3.2 3.5 4.3 4.8 5.1]'  InternalRulePriority=Speed  RndMeth=Simplest
      settings: InputPortMap=u0,u1
  Fan Area [m^2] : Gain  Gain=vehicleThermal.fan_area
  Max Fan : Gain  Gain=14.4
  Simulink-PS Converter4 : nesl_utility/Simulink-PS Converter  PhysicalDomain=network_engine_domain  SubClassName=ps_input  LeftPortType=input  RightPortType=output  PseudoPeriodic=off  Frequencies=[]  NoiseDistribution=none  NoiseParameters=[]  Unit=m^3/s  AffineConversion=off  FilteringAndDerivatives=provide  SimscapeFilterOrder=1  InputFilterTimeConstant=0.001  UdotUserProvided=0
  Transfer Fcn : TransferFcn  Denominator=[5 1]
  disp : PMIOPort  Side=Right
  wires:
  Max Fan/1 -> Air Speed Table [m/s]/2
  Transfer Fcn/1 -> Fan Area [m^2]/1
  Air Speed Table [m/s]/1 -> Transfer Fcn/1
  FanCtrl/1 -> Max Fan/1
  VehSpd/1 -> Air Speed Table [m/s]/1
  Fan Area [m^2]/1 -> Simulink-PS Converter4/1
  connections:
  disp/RConn1 -- Simulink-PS Converter4/RConn1

== system VehicleElectroThermal/Radiator/Subsystem ==
  s : Inport
  Bus Selector : BusSelector  OutputSignals=Env,VehSpd,cmdFan
  Bus Selector1 : BusSelector  OutputSignals=Tenv,Penv,RHenv,CO2env
  T : Outport
  p : Outport  Port=2
  RH : Outport  Port=3
  CO2 : Outport  Port=4
  VehSpd : Outport  Port=5
  cmdFan : Outport  Port=6
  wires:
  Bus Selector1/4 -> CO2/1  "<CO2env>"
  Bus Selector/2 -> VehSpd/1  "<VehSpd>"
  Bus Selector1/1 -> T/1  "<Tenv>"
  s/1 -> Bus Selector/1
  Bus Selector1/2 -> p/1  "<Penv>"
  Bus Selector/1 -> Bus Selector1/1  "<Env>"
  Bus Selector/3 -> cmdFan/1  "<cmdFan>"
  Bus Selector1/3 -> RH/1  "<RHenv>"

== system VehicleElectroThermal/Rear Motor (EM2)/Emotor Input ==
  TrqCmd : Inport
  " Batt" : Inport  Port=2
  Bus Creator : BusCreator  Inputs=3
  Bus Selector3 : BusSelector  OutputSignals=Relay.RelayDchg,BattSensor.BatVolt
  Constant : Constant
  Constant1 : Constant  Value=0
  Gain : Gain
  Switch : Switch  Criteria=u2 > Threshold  SaturateOnIntegerOverflow=off  InputSameDT=off
  EMctl : Outport
  wires:
  Gain/1 -> Bus Creator/3  "BatVolt"
  Bus Selector3/2 -> Gain/1  "<BatVolt>"
  Bus Creator/1 -> EMctl/1
  " Batt"/1 -> Bus Selector3/1
  Bus Selector3/1 -> Switch/2  "<RelayDchg>"
  Constant/1 -> Switch/3
  Constant1/1 -> Switch/1
  Switch/1 -> Bus Creator/2  "fault"
  TrqCmd/1 -> Bus Creator/1  "EMtrq"

== system VehicleElectroThermal/Rear Motor (EM2)/Emotor Output ==
  S : Inport
  Bus Selector1 : BusSelector  OutputSignals=Current,Volt
  Constant : Constant  Value=3600
  Divide : Product  Inputs=*/
  Integrator : Integrator
  Product : Product
  EM2 : Outport
  E : Outport  Port=2
  wires:
  Bus Selector1/1 -> Product/1  "<Current>"
  Bus Selector1/2 -> Product/2  "<Volt>"
  S/1 -> Bus Selector1/1, EM2/1  "EM2sensor"
  Product/1 -> Integrator/1
  Integrator/1 -> Divide/1
  Constant/1 -> Divide/2
  Divide/1 -> E/1  "EM2energy"

== system VehicleElectroThermal/Rear Motor (EM2)/Inverter PM Thermal ==
  IGBTlossTable : fl_lib/Physical Signals/Lookup Tables/PS Lookup Table (3D)  x1=electricDrive.motor_loss_map.spMat rpm  x2=electricDrive.motor_loss_map.tqMat N*m  x3=[25,125, 175]+273.15 K  f=electricDrive.inverter_loss_map.lossMatIgbt  interp_method=simscape.enum.interpolation.linear  extrap_method=simscape.enum.extrapolation.linear
      settings: InternalSimscapePortConfiguration="{\"Bottom\":[],\"Left\":[{\"id\":\"I1\",\"label\":\"x1\",\"type\":\"input\"},{\"id\":\"I2\",\"label\":\"x2\",\"type\":\"input\"},{\"id\":\"I3\",\"label\":\"x3\",\"type\":\"input\"}],\"Right\":[{\"id\":\"O\",\"label\":\"f\",\"type\":\"output\"}],\"Top\":[]}"
  PM Cauer thermal : Subsystem
      settings: PortSchema="{\"entries\":[{\"content\":{\"sides\":[{\"content\":{\"connectorIds\":[\"LConn1\"]},\"type\":\"ConnectorPlacement.EquallySpacedRectSide\",\"uuid\":\"c466717f-a559-4c42-b6dd-2de508982627\"},{\"content\":{\"connectorIds\":[\"RConn1\",\"RConn2\",\"RConn3\"],\"side\":\"RIGHT\"},\"type\":\"ConnectorPlacement.EquallySpacedRectSide\",\"uuid\":\"5a44429a-0c01-47a4-96c4-89a03d92af2a\"},{\"content\":{\"connectorIds\":[],\"side\":\"TOP\"},\"type\":\"ConnectorPlacement.EquallySpacedRectSide\",\"uuid\":\"592797f6-2176-45a1-8a5a-ffba72eaaa30\"},{\"content\":{\"connectorIds\":[\"RConn4\",\"RConn5\"],\"side\":\"BOTTOM\"},\"type\":\"ConnectorPlacement.EquallySpacedRectSide\",\"uuid\":\"45f39216-5c54-48d4-857b-159bfbffda40\"}]},\"type\":\"ConnectorPlacement.EquallySpacedConnector\",\"uuid\":\"8211d252-7bec-4c59-be39-60a0fcf206ce\"}],\"packageUris\":[\"http://schema.mathworks.com/mf0/Connector/R2020b\"],\"version\":\"1.0\"}"
  diodeLossTable : fl_lib/Physical Signals/Lookup Tables/PS Lookup Table (3D)  x1=electricDrive.motor_loss_map.spMat rpm  x2=electricDrive.motor_loss_map.tqMat N*m  x3=[25,125, 175]+273.15 K  f=electricDrive.inverter_loss_map.lossMatDiode  interp_method=simscape.enum.interpolation.linear  extrap_method=simscape.enum.extrapolation.linear
      settings: InternalSimscapePortConfiguration="{\"Bottom\":[],\"Left\":[{\"id\":\"I1\",\"label\":\"x1\",\"type\":\"input\"},{\"id\":\"I2\",\"label\":\"x2\",\"type\":\"input\"},{\"id\":\"I3\",\"label\":\"x3\",\"type\":\"input\"}],\"Right\":[{\"id\":\"O\",\"label\":\"f\",\"type\":\"output\"}],\"Top\":[]}"
  Vliq : PMIOPort  Side=Left
  Motor RPM : PMIOPort  Port=2  Side=Left
  Motor Torque : PMIOPort  Port=3  Side=Left
  H : PMIOPort  Port=4  Side=Right
  connections:
  PM Cauer thermal/RConn5 -- IGBTlossTable/LConn3
  PM Cauer thermal/RConn2 -- diodeLossTable/LConn3
  IGBTlossTable/LConn2 -- Motor Torque/RConn1 -- diodeLossTable/LConn2
  IGBTlossTable/LConn1 -- diodeLossTable/LConn1 -- Motor RPM/RConn1
  Vliq/RConn1 -- PM Cauer thermal/RConn4
  diodeLossTable/RConn1 -- PM Cauer thermal/RConn1
  IGBTlossTable/RConn1 -- PM Cauer thermal/RConn3
  H/RConn1 -- PM Cauer thermal/LConn1

== system VehicleElectroThermal/Rear Motor (EM2)/SC1 ==
  Absolute Reference (TL) : fl_lib/Thermal Liquid/Elements/Absolute Reference (TL)
  Pressure & Temperature Sensor (TL) : fl_lib/Thermal Liquid/Sensors/Pressure & Temperature Sensor (TL)  reference=foundation.enum.MeasurementReference.difference  pressure=true  pressure_spec=foundation.enum.PressureMeasementSpec.Absolute  temperature=true
      settings: InternalSimscapePortConfiguration="{\"Bottom\":[{\"id\":\"T\",\"label\":\"T\",\"type\":\"output\"}],\"Left\":[{\"id\":\"A\",\"label\":\"A\",\"type\":\"foundation.thermal_liquid.thermal_liquid\"}],\"Right\":[{\"id\":\"B\",\"label\":\"B\",\"type\":\"foundation.thermal_liquid.thermal_liquid\"},{\"id\":\"P\",\"label\":\"P\",\"type\":\"output\"}],\"Top\":[]}"
  Volumetric Flow Rate Sensor (TL) : fl_lib/Thermal Liquid/Sensors/Flow Rate Sensor (TL)  mass_flow_measure=false  volumetric_flow_measure=true  energy_flow_measure=false
      settings: InternalSimscapePortConfiguration="{\"Bottom\":[],\"Left\":[{\"id\":\"A\",\"label\":\"A\",\"type\":\"foundation.thermal_liquid.thermal_liquid\"}],\"Right\":[{\"id\":\"B\",\"label\":\"B\",\"type\":\"foundation.thermal_liquid.thermal_liquid\"},{\"id\":\"V\",\"label\":\"V\",\"type\":\"output\"}],\"Top\":[]}"
  B : PMIOPort  Side=Left
  A : PMIOPort  Port=2  Side=Right
  m3/s : PMIOPort  Port=3  Side=Right
  connections:
  Volumetric Flow Rate Sensor (TL)/RConn2 -- m3/s/RConn1
  Absolute Reference (TL)/LConn1 -- Pressure & Temperature Sensor (TL)/RConn1
  Volumetric Flow Rate Sensor (TL)/LConn1 -- B/RConn1
  Volumetric Flow Rate Sensor (TL)/RConn1 -- A/RConn1 -- Pressure & Temperature Sensor (TL)/LConn1

== system VehicleElectroThermal/Rear Motor (EM2)/m3//s to m//s ==
  note: Q=Av
  Coolant Area : fl_lib/Physical Signals/Sources/PS Constant  constant=4 * pi * vehicleThermal.coolant_channel_D^2 / 4 m^2
  PS Divide : fl_lib/Physical Signals/Functions/PS Divide
  PS Saturation : fl_lib/Physical Signals/Nonlinear Operators/PS Saturation  upper_limit=10 m/s  lower_limit=1e-6 m/s
  "  " : PMIOPort  Side=Left
  Vliq : PMIOPort  Port=2  Side=Right
  connections:
  PS Divide/RConn1 -- PS Saturation/LConn1
  PS Saturation/RConn1 -- Vliq/RConn1
  "  "/RConn1 -- PS Divide/LConn1
  PS Divide/LConn2 -- Coolant Area/RConn1

== system VehicleElectroThermal/Chiller/Chiller Subsystem/Chiller Demand ==
  No current : fl_lib/Physical Signals/Sources/PS Constant  constant=0 A
  PS Abs : fl_lib/Physical Signals/Nonlinear Operators/PS Abs
      settings: InternalSimscapePortConfiguration="{\"Bottom\":[],\"Left\":[{\"id\":\"I\",\"label\":\"\",\"type\":\"input\"}],\"Right\":[{\"id\":\"O\",\"label\":\"\",\"type\":\"output\"}],\"Top\":[]}"
  PS Add : fl_lib/Physical Signals/Functions/PS Add
  PS Divide : fl_lib/Physical Signals/Functions/PS Divide
  PS Switch : fl_lib/Physical Signals/Nonlinear Operators/PS Switch  Threshold=0.5
      settings: InternalSimscapePortConfiguration="{\"Bottom\":[],\"Left\":[{\"id\":\"I1\",\"label\":\"\",\"type\":\"input\"},{\"id\":\"I2\",\"label\":\"\",\"type\":\"input\"},{\"id\":\"I3\",\"label\":\"\",\"type\":\"input\"}],\"Right\":[{\"id\":\"O\",\"label\":\"\",\"type\":\"output\"}],\"Top\":[]}"
  Zero Divide Protection : fl_lib/Physical Signals/Sources/PS Constant  constant=1 V
  Volt : PMIOPort  Side=Left
  BatSt : PMIOPort  Port=2  Side=Left
  P : PMIOPort  Port=3  Side=Left
  I : PMIOPort  Port=4  Side=Right
  connections:
  I/RConn1 -- PS Switch/RConn1
  P/RConn1 -- PS Abs/LConn1
  PS Abs/RConn1 -- PS Divide/LConn1
  PS Add/LConn2 -- Zero Divide Protection/RConn1
  PS Add/RConn1 -- PS Divide/LConn2
  BatSt/RConn1 -- PS Switch/LConn2
  PS Switch/LConn1 -- PS Divide/RConn1
  PS Add/LConn1 -- Volt/RConn1
  No current/RConn1 -- PS Switch/LConn3
